simulink model "JulyTestV1"  (Simulink 7.3)
settings: Solver=FixedStepDiscrete  StartTime=0.0  StopTime=inf  FixedStep=0.1  MaxStep=0.2  RelTol=1e-3
libraries: dspmtrx3 x3, simulink x2, vipstatistics x2, dspstat3 x2
(part 1 of 2)
settings Model: Creator=gclayton  LastModifiedBy=wildcat
settings DebuggingCC: InheritedTsInSrcMsg=none
settings RTWCC: SystemTargetFile=rlnx.tlc  GenCodeOnly=on  TemplateMakefile=rlnx_ubuntu.tmf  Description=Linux Real-Time Target  ProcessScript=rlnx_make_rtw_hook
settings RTWCC: CustomInclude=|
  | /usr/local/include/opencv/
  | /usr/local/include/
settings CodeAppCC: GenerateComments=off  SimulinkBlockComments=off
settings STFCustomTargetCC: ModelReferenceCompliant=off  MatFileLogging=on  SystemTargetFile=rlnx.tlc
settings GRTTargetCC: ModelReferenceCompliant=off  ParMdlRefBuildCompliant=off  CompOptLevelCompliant=off
settings CustomProperty: DataType=string  Value="-lm -ldl /usr/local/lib/libopencv_highgui.so.2.4 /usr/local/lib/libopencv_core.so.2.4 /usr/local/lib/libopencv_imgproc.so.2.4  -lc_urg -lc_urg_connection -lc_urg_system -lphidget21"
settings EnumStrPairs: String=PC

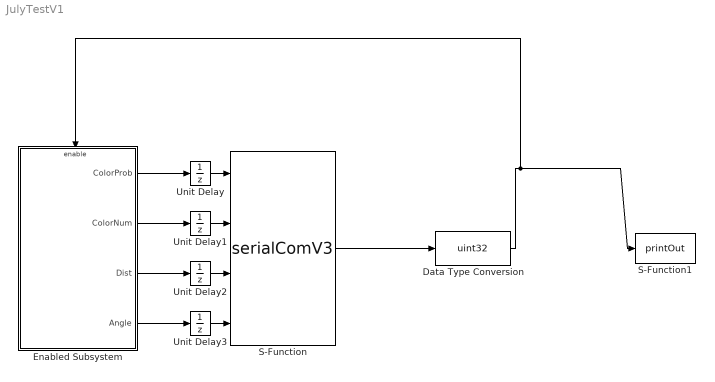
== system JulyTestV1 ==
  Data Type Conversion : DataTypeConversion  OutDataTypeMode=uint32  OutDataType=fixdt(1, 16)  OutScaling=2^0  OutDataTypeStr=uint32
  Enabled Subsystem : Subsystem  TreatAsAtomicUnit=on
  S-Function : S-Function  FunctionName=serialComV3  EnableBusSupport=off
  S-Function1 : S-Function  FunctionName=printOut  EnableBusSupport=off
  Unit Delay : UnitDelay  SampleTime=-1
  Unit Delay1 : UnitDelay  X0=int32(0)  SampleTime=-1
  Unit Delay2 : UnitDelay  X0=int32(0)  SampleTime=-1
  Unit Delay3 : UnitDelay  X0=int32(0)  SampleTime=-1
  wires:
  S-Function/1 -> Data Type Conversion/1
  Data Type Conversion/1 -> S-Function1/1, Enabled Subsystem/Enable
  Enabled Subsystem/1(ColorProb) -> Unit Delay/1
  Enabled Subsystem/2(ColorNum) -> Unit Delay1/1
  Enabled Subsystem/3(Dist) -> Unit Delay2/1
  Enabled Subsystem/4(Angle) -> Unit Delay3/1
  Unit Delay/1 -> S-Function/1
  Unit Delay1/1 -> S-Function/2
  Unit Delay2/1 -> S-Function/3
  Unit Delay3/1 -> S-Function/4

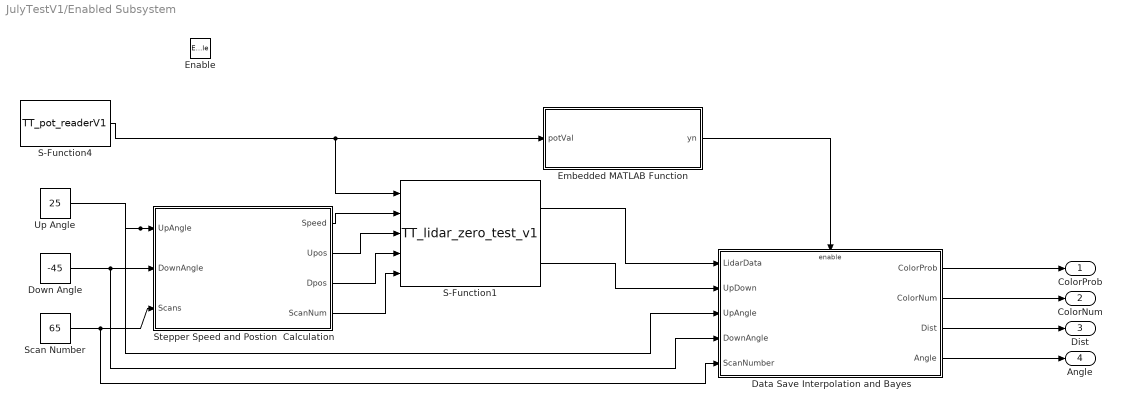
== system JulyTestV1/Enabled Subsystem ==
  Enable : EnablePort
  Data Save Interpolation and Bayes : Subsystem  TreatAsAtomicUnit=on
  Down Angle : Constant  Value=-45  OutDataType=fixdt(1, 16)  OutScaling=2^0
  Embedded MATLAB Function : Stateflow chart
  S-Function1 : S-Function  FunctionName=TT_lidar_zero_test_v1  EnableBusSupport=off
  S-Function4 : S-Function  FunctionName=TT_pot_readerV1  EnableBusSupport=off
  Scan Number : Constant  Value=65  OutDataType=fixdt(1, 16)  OutScaling=2^0
  Stepper Speed and Postion  Calculation : Stateflow chart
  Up Angle : Constant  Value=25  OutDataType=fixdt(1, 16)  OutScaling=2^0
  ColorProb : Outport  OutDataType=fixdt(1, 16)  OutScaling=2^0
  ColorNum : Outport  Port=2  OutDataType=fixdt(1, 16)  OutScaling=2^0
  Dist : Outport  Port=3  OutDataType=fixdt(1, 16)  OutScaling=2^0
  Angle : Outport  Port=4  OutDataType=fixdt(1, 16)  OutScaling=2^0
  wires:
  S-Function4/1 -> S-Function1/1, Embedded MATLAB Function/1(potVal)
  Scan Number/1 -> Stepper Speed and Postion  Calculation/3(Scans), Data Save Interpolation and Bayes/5(ScanNumber)
  Down Angle/1 -> Stepper Speed and Postion  Calculation/2(DownAngle), Data Save Interpolation and Bayes/4(DownAngle)
  Up Angle/1 -> Stepper Speed and Postion  Calculation/1(UpAngle), Data Save Interpolation and Bayes/3(UpAngle)
  Stepper Speed and Postion  Calculation/1(Speed) -> S-Function1/2
  Stepper Speed and Postion  Calculation/2(Upos) -> S-Function1/3
  Stepper Speed and Postion  Calculation/3(Dpos) -> S-Function1/4
  Stepper Speed and Postion  Calculation/4(ScanNum) -> S-Function1/5
  Embedded MATLAB Function/1(yn) -> Data Save Interpolation and Bayes/Enable
  S-Function1/1 -> Data Save Interpolation and Bayes/1(LidarData)
  S-Function1/2 -> Data Save Interpolation and Bayes/2(UpDown)
  Data Save Interpolation and Bayes/1(ColorProb) -> ColorProb/1
  Data Save Interpolation and Bayes/2(ColorNum) -> ColorNum/1
  Data Save Interpolation and Bayes/3(Dist) -> Dist/1
  Data Save Interpolation and Bayes/4(Angle) -> Angle/1

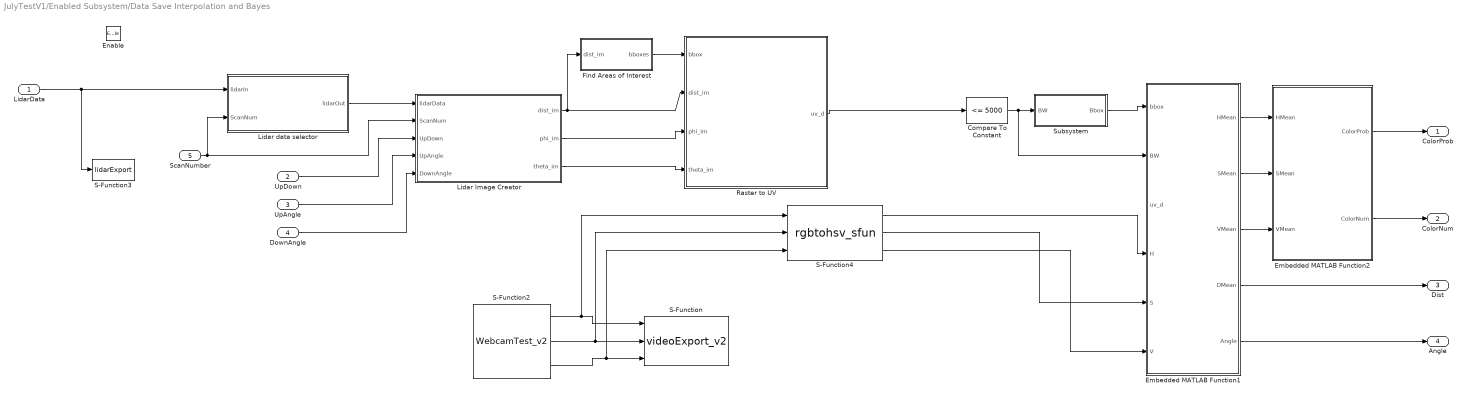
== system JulyTestV1/Enabled Subsystem/Data Save Interpolation and Bayes ==
  LidarData : Inport  OutDataType=fixdt(1, 16)  OutScaling=2^0
  UpDown : Inport  Port=2  OutDataType=fixdt(1, 16)  OutScaling=2^0
  UpAngle : Inport  Port=3  OutDataType=fixdt(1, 16)  OutScaling=2^0
  DownAngle : Inport  Port=4  OutDataType=fixdt(1, 16)  OutScaling=2^0
  ScanNumber : Inport  Port=5  OutDataType=fixdt(1, 16)  OutScaling=2^0
  Enable : EnablePort
  Compare To Constant : simulink/Logic and Bit Operations/Compare To Constant  SystemSampleTime=-1  relop=<=  const=5000  LogicOutDataTypeMode=boolean  ZeroCross=off
  Embedded MATLAB Function1 : Stateflow chart
  Embedded MATLAB Function2 : Stateflow chart
  Find Areas of Interest : Subsystem
  Lidar Image Creator : Stateflow chart
  Lidar data selector : Stateflow chart
  Raster to UV : Stateflow chart
  S-Function : S-Function  FunctionName=videoExport_v2  EnableBusSupport=off
  S-Function2 : S-Function  FunctionName=WebcamTest_v2  EnableBusSupport=off
  S-Function3 : S-Function  FunctionName=lidarExport  EnableBusSupport=off
  S-Function4 : S-Function  FunctionName=rgbtohsv_sfun  EnableBusSupport=off
  Subsystem : Subsystem
  ColorProb : Outport  OutDataType=fixdt(1, 16)  OutScaling=2^0
  ColorNum : Outport  Port=2  OutDataType=fixdt(1, 16)  OutScaling=2^0
  Dist : Outport  Port=3  OutDataType=fixdt(1, 16)  OutScaling=2^0
  Angle : Outport  Port=4  OutDataType=fixdt(1, 16)  OutScaling=2^0
  wires:
  S-Function2/3 -> S-Function/3, S-Function4/3
  S-Function2/2 -> S-Function/2, S-Function4/2
  S-Function2/1 -> S-Function/1, S-Function4/1
  LidarData/1 -> S-Function3/1, Lidar data selector/1(lidarIn)
  ScanNumber/1 -> Lidar data selector/2(ScanNum), Lidar Image Creator/2(ScanNum)
  Lidar data selector/1(lidarOut) -> Lidar Image Creator/1(lidarData)
  UpDown/1 -> Lidar Image Creator/3(UpDown)
  UpAngle/1 -> Lidar Image Creator/4(UpAngle)
  DownAngle/1 -> Lidar Image Creator/5(DownAngle)
  Lidar Image Creator/1(dist_im) -> Raster to UV/2(dist_im), Find Areas of Interest/1(dist_im)
  Lidar Image Creator/2(phi_im) -> Raster to UV/3(phi_im)
  Lidar Image Creator/3(theta_im) -> Raster to UV/4(theta_im)
  Find Areas of Interest/1(bboxes) -> Raster to UV/1(bbox)
  Compare To Constant/1 -> Subsystem/1(BW), Embedded MATLAB Function1/2(BW)
  Subsystem/1(Bbox) -> Embedded MATLAB Function1/1(bbox)
  Embedded MATLAB Function1/3(VMean) -> Embedded MATLAB Function2/3(VMean)
  Embedded MATLAB Function1/2(SMean) -> Embedded MATLAB Function2/2(SMean)
  Embedded MATLAB Function1/1(HMean) -> Embedded MATLAB Function2/1(HMean)
  Raster to UV/1(uv_d) -> Compare To Constant/1
  S-Function4/1 -> Embedded MATLAB Function1/4(H)
  S-Function4/2 -> Embedded MATLAB Function1/5(S)
  S-Function4/3 -> Embedded MATLAB Function1/6(V)
  Embedded MATLAB Function2/1(ColorProb) -> ColorProb/1
  Embedded MATLAB Function2/2(ColorNum) -> ColorNum/1
  Embedded MATLAB Function1/4(DMean) -> Dist/1
  Embedded MATLAB Function1/5(Angle) -> Angle/1

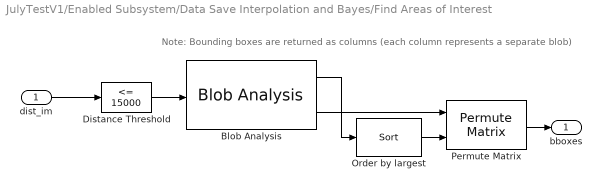
== system JulyTestV1/Enabled Subsystem/Data Save Interpolation and Bayes/Find Areas of Interest ==
  note: Note: Bounding boxes are returned as columns (each column represents a separate blob)
  dist_im : Inport  OutDataType=fixdt(1, 16)  OutScaling=2^0
  Blob Analysis : vipstatistics/Blob Analysis  DialogController=vipDDGCreate  DialogControllerArgs=DataTag0  area=on  centroid=off  bBox=on  majorAxis=off  minorAxis=off  angle=off  eccentricity=off  equivDiameterSq=off  extent=off  perimeter=off  maxBlobs=8  warnIfNumBlobsExceeded=on  isCount=off  useMinArea=off  minArea=0  useMaxArea=off  maxArea=intmax('uint32')  excludeBorderBlob=off  outDT=double  isOutVarDim=off  isFill=on  fillValues=-1  conn=8  isLabel=off  outputMode=Binary point scaling  outputWordLength=32  outputFracLength=16  firstCoeffMode=Binary point scaling  firstCoeffWordLength=16  firstCoeffFracLength=14  secondCoeffMode=Binary point scaling  secondCoeffWordLength=32  secondCoeffFracLength=16  accumMode=Binary point scaling  accumWordLength=32  accumFracLength=0  prodOutputMode=Binary point scaling  prodOutputWordLength=32  prodOutputFracLength=16  roundingMode=Floor  overflowMode=off
  Distance Threshold : simulink/Logic and Bit Operations/Compare To Constant  SystemSampleTime=-1  relop=<=  const=15000  LogicOutDataTypeMode=boolean  ZeroCross=off
  Order by largest : dspstat3/Sort  DialogController=dspDDGCreate  DialogControllerArgs=DataTag1  otype=Index  dir=Descending  sortAlg=Quick sort  roundingMode=Floor  overflowMode=off
  Permute Matrix : dspmtrx3/Permute Matrix  mode=Columns  ZeroOneIdxMode=One-based  errmode=Clip index  checkDims=off
  bboxes : Outport  OutDataType=fixdt(1, 16)  OutScaling=2^0
  wires:
  dist_im/1 -> Distance Threshold/1
  Distance Threshold/1 -> Blob Analysis/1
  Blob Analysis/2 -> Permute Matrix/1
  Order by largest/1 -> Permute Matrix/2
  Blob Analysis/1 -> Order by largest/1
  Permute Matrix/1 -> bboxes/1

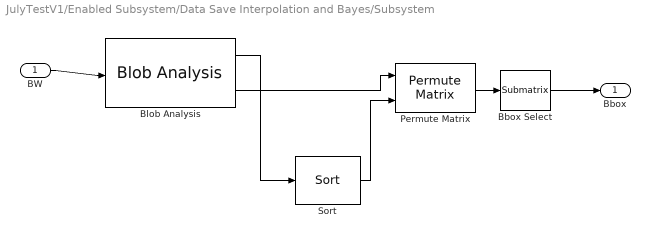
== system JulyTestV1/Enabled Subsystem/Data Save Interpolation and Bayes/Subsystem ==
  BW : Inport  OutDataType=fixdt(1, 16)  OutScaling=2^0
  Bbox Select : dspmtrx3/Submatrix  RowSpan=One row  RowStartMode=First  RowStartIndex=1  RowEndMode=Last  RowEndIndex=1  ColSpan=All columns  ColStartMode=First  ColStartIndex=1  ColEndMode=Last  ColEndIndex=1
  Blob Analysis : vipstatistics/Blob Analysis  DialogController=vipDDGCreate  DialogControllerArgs=DataTag2  area=on  centroid=off  bBox=on  majorAxis=off  minorAxis=off  angle=off  eccentricity=off  equivDiameterSq=off  extent=off  perimeter=off  maxBlobs=20  warnIfNumBlobsExceeded=on  isCount=off  useMinArea=on  minArea=20  useMaxArea=off  maxArea=intmax('uint32')  excludeBorderBlob=off  outDT=double  isOutVarDim=off  isFill=on  fillValues=-1  conn=8  isLabel=off  outputMode=Binary point scaling  outputWordLength=32  outputFracLength=16  firstCoeffMode=Binary point scaling  firstCoeffWordLength=16  firstCoeffFracLength=14  secondCoeffMode=Binary point scaling  secondCoeffWordLength=32  secondCoeffFracLength=16  accumMode=Binary point scaling  accumWordLength=32  accumFracLength=0  prodOutputMode=Binary point scaling  prodOutputWordLength=32  prodOutputFracLength=16  roundingMode=Floor  overflowMode=off
  Permute Matrix : dspmtrx3/Permute Matrix  mode=Columns  ZeroOneIdxMode=One-based  errmode=Clip index  checkDims=off
  Sort : dspstat3/Sort  DialogController=dspDDGCreate  DialogControllerArgs=DataTag3  otype=Index  dir=Descending  sortAlg=Quick sort  roundingMode=Floor  overflowMode=off
  Bbox : Outport  OutDataType=fixdt(1, 16)  OutScaling=2^0
  wires:
  BW/1 -> Blob Analysis/1
  Blob Analysis/1 -> Sort/1
  Sort/1 -> Permute Matrix/2
  Blob Analysis/2 -> Permute Matrix/1
  Permute Matrix/1 -> Bbox Select/1
  Bbox Select/1 -> Bbox/1

== matlab function Enabled Subsystem/Stepper Speed and Postion Calculation ==
  data: UpAngle input double; Speed output double; DownAngle input double; Scans input double; Upos output double; Dpos output double; ScanNum output double
function [Speed,Upos,Dpos,ScanNum] = stepper_calc(UpAngle,DownAngle,Scans)

% This function inputs desired positive and negative scan angles
% and desired number of scans and outputs results positions for
% the stepper and the required speed of the stepper motor to properly
% move so the desired number of scans is obtained over the course of
% the motion of the stepper

% Scan Number requires no change
ScanNum = Scans;

% Transformation of angle to stepper position obtained from stepper calibration
% Output must be an integer
% 57 is added or subtracted due to wobble of gimbal system
Upos = round(UpAngle*1036/45)-57;
Dpos = round(DownAngle*1036/45)+57;

% Transformation of speed based 
% Output must be an interger
Speed = round(abs(UpAngle-DownAngle) * (1214/90) * 65/Scans);

== matlab function Enabled Subsystem/Embedded MATLAB Function ==
  data: potVal input double; yn output double
function yn = check_pot_val(potVal)
%#eml

% Pot value may initially be zero.
% Check for this and output a 1 or zero to 
% control whether the rest of model runs
if (potVal == 0)
    yn = 0;
else
    yn = 1;
end

== matlab function Enabled Subsystem/Data Save Interpolation and Bayes/Lidar data selector ==
  data: lidarIn input double; lidarOut output double; ScanNum input double
function lidarOut = data_selector(lidarIn,ScanNum)
% Lidar data is always input as a 1x70200 matrix.
% If Scan Number is less than 65 some of this data may be blank
% Select only the parts of the matrix where data has been collected

% FullLength = 1080*65;
% DataLength =  1080*ScanNum;
% lidarOut = zeros(1,FullLength);

ClosePts = (lidarIn < 3);
lidarOut = lidarIn + 30000*ClosePts;

% for i = 1:DataLength
%     if (lidarIn(i) < 3)
%         lidarIn(i) = 30000;
%     end
%     lidarOut(i) = lidarIn(i);
% end

%lidarOut = lidarIn(1,1:DataLength);

== matlab function Enabled Subsystem/Data Save Interpolation and Bayes/Lidar Image Creator ==
  data: lidarData input double; ScanNum input double; dist_im output double; phi_im output double; theta_im output double; UpDown input double; UpAngle input double; DownAngle input double
function [dist_im, phi_im, theta_im] = image_creator(lidarData,ScanNum,UpDown,UpAngle,DownAngle)
%#eml

% Define variables based on gimbal system and scan pattern
FullLength = 1080*65;
DataLength = 1080*ScanNum;
h = 36.3;

% Define Data sizes
phim = zeros(1,FullLength);
thetam = zeros(1,FullLength);
distm = zeros(1,FullLength);
dist_im = zeros(65,540);
phi_im = zeros(65,540);
theta_im = zeros(65,540);


%Define phi_rad: angles corresponding to one lidar scan
l = 1:1080;
phi_rad = (-45 + 0.25*l)*pi/180;

% Repeat phim for number of scans
for i = 1:ScanNum
        
    for j = 1 : 1080
        phi_val = 1080*(i-1) + j;
        phim(1,phi_val) = phi_rad(1,j);
    end
end

% Theta changes from -45 to 45 degrees over the duration of the scan
theta_min = DownAngle*pi/180;
theta_max = UpAngle*pi/180;
theta_step = (theta_max - theta_min)/DataLength;

for i1 = 1:DataLength
    if (UpDown == 0)
        thetam(i1) = theta_max - theta_step*(i1-1);
    elseif (UpDown == 1)
        thetam(i1) = theta_min + theta_step*(i1-1);
    end
end

% Distance matrix is directly from lidar data
distm = lidarData';


% Create images for distance, phi, and theta
for i2 = 1:ScanNum
    for j2 = 1:540
        dist_im(i2,j2) = distm(1, 270+j2 + 1080*(i2-1));
        phi_im(i2,j2) = phim(1, 270+j2 + 1080*(i2-1));
        theta_im(i2,j2) = thetam(1, 270+j2 + 1080*(i2-1));
    end
    
end

== matlab function Enabled Subsystem/Data Save Interpolation and Bayes/Raster to UV ==
  data: bbox input double; uv_d output double; dist_im input double; phi_im input double; theta_im input double
function uv_d  = fcn(bbox,dist_im,phi_im,theta_im)
% Written by Anderson Lebbad on July 3, 2014
% Last Edited:
%
% This function transforms the lidar raster image into u,v coordinates,
% with an xyz transformation and change of perspective from the lidar to
% the camera

%% Set Variables

% Find the number of valid bounding boxes
numBBox = 8 - sum(bbox(1,:) == -1);

beyondRange = 30000;
uv_d = beyondRange*ones(480,640);

% Initialize size of X,Y and Z matrices
X = zeros(size(dist_im));
Y = zeros(size(dist_im));
Z = zeros(size(dist_im));
Xc = zeros(size(dist_im));
Yc = zeros(size(dist_im));
Zc = zeros(size(dist_im));
Xn = zeros(size(dist_im));
Yn = zeros(size(dist_im));
Xp = zeros(size(dist_im));
Yp = zeros(size(dist_im));
Dp = zeros(size(dist_im));
r2 = zeros(size(dist_im));
r6 = zeros(size(dist_im));
Xd = zeros(size(dist_im));
Yd = zeros(size(dist_im));

% Height of the lidar on the gimbal
h = 36.3;

% Translation vector (in millimeters)
t = [24; -113; 38];

% Rotation angles
phi = (-90+6)*pi/180;
theta = 0*pi/180;

% Rotation about the x-axis
Rx = [1 0 0; 0 cos(phi) sin(phi); 0 -sin(phi) cos(phi)];
% Followed by rotation about the y-axis
R = [cos(theta) 0 -sin(theta); 0 1 0; sin(theta) 0 cos(theta)]*Rx;

% Transformation matrix
T = [R t];

% Radial Distortions
RadDist = [0.069102182282360,-0.154608606024690,0.020241053576861];

% Intrinsic Matrix
K = [5.548581600685270e+02,0,0;0,5.523116000564020e+02,0;3.135858904821101e+02,2.190392333699872e+02,1];
KK = K';

% Iterate filling points into XYZ matrices for each valid bbox
for i = 1:numBBox
    
    % Initialize values for looped info
    minXp = 10000;
    maxXp = -10000;
    minYp = 10000;
    maxYp = -10000;
    
    % Find region to fill
    minX = bbox(1,i);
    maxX = minX + bbox(3,i) - 1;
    minY = bbox(2,i);
    maxY = minY + bbox(4,i) - 1;
    
    % Loop for each pixel in the bounding box
    for j = minX:maxX
        for k = minY:maxY
            % Convert to XYZ
            X(k,j) = dist_im(k,j).*cos(phi_im(k,j));
            Y(k,j) = dist_im(k,j).*sin(phi_im(k,j)).*cos(theta_im(k,j))-h.*sin(theta_im(k,j));
            Z(k,j) = dist_im(k,j).*sin(phi_im(k,j)).*sin(theta_im(k,j))+h.*cos(theta_im(k,j));
            
            % Transformation to camera coordinate frame
            Xc(k,j) = T(1,1)*X(k,j)+T(1,2)*Y(k,j)+T(1,3)*Z(k,j)+T(1,4);
            Yc(k,j) = T(2,1)*X(k,j)+T(2,2)*Y(k,j)+T(2,3)*Z(k,j)+T(2,4);
            Zc(k,j) = T(3,1)*X(k,j)+T(3,2)*Y(k,j)+T(3,3)*Z(k,j)+T(3,4);
            
            % Normalize Coordinates
            Xn(k,j) = Xc(k,j)./Zc(k,j);
            Yn(k,j) = Yc(k,j)./Zc(k,j);
            
            % Calculate Distance to each point from camera
            Dp(k,j) = sqrt(Xc(k,j).^2+Yc(k,j).^2+Zc(k,j).^2);
            
            % Radial Vectors
            r2(k,j) = Xn(k,j).^2+Yn(k,j).^2;
            r6(k,j) = r2(k,j).^3;
            
            % Distorted Coodinates
            Xd(k,j) = Xn(k,j).*(1+RadDist(1).*r2(k,j)+RadDist(3).*r6(k,j));
            Yd(k,j) = Yn(k,j).*(1+RadDist(1).*r2(k,j)+RadDist(3).*r6(k,j));
            
            % Pixel Coordinates
            Xp(k,j) = KK(1,1)*Xd(k,j)+KK(1,2)*Yd(k,j)+KK(1,3);
            Yp(k,j) = KK(2,1)*Xd(k,j)+KK(2,2)*Yd(k,j)+KK(2,3);
            
            % Find area the blob is bound by in the image coordinates
            minXp = ceil(min(Xp(k,j),minXp));
            maxXp = floor(max(Xp(k,j),maxXp));
            minYp = ceil(min(Yp(k,j),minYp));
            maxYp = floor(max(Yp(k,j),maxYp));
        end
    end
    
    % Check to make sure blob is (at least partially) within image frame
    if (minXp < 640) && (maxXp > 1) && (minYp < 480) && (maxYp > 1)
        
        % Set interpolation vectors to not exceed frame
        minXp = max(minXp,1);
        maxXp = min(maxXp,640);
        minYp = max(minYp,1);
        maxYp = min(maxYp,480);
        
        % Run interpolation over bounded region
        for j3 = minXp:maxXp
            for k3 = minYp:maxYp
                
                % Initialize values
                l1normSmall = 1000;
                uPt = int32(1);
                vPt = int32(1);
                
                % Loop for each pixel in original bounding box
                for j2 = minX:maxX
                    for k2 = minY:maxY
                        
                        % L1 Norm for nearest neighbor interpolation
                        l1norm = abs(Xp(k2,j2)-j3)+abs(Yp(k2,j2)-k3);
                        
                        % Check against previously smallest L1 norm
                        if l1norm < l1normSmall
                            % Replace previous value with current value
                            l1normSmall = l1norm;
                            uPt = j2;
                            vPt = k2;
                        end
                    end
                end
                
                % Use pointer array to assign depth values into output frame
                uv_d(k3,j3) = Dp(uPt,vPt);
                
            end
        end
    end
end

end

== matlab function Enabled Subsystem/Data Save Interpolation and Bayes/Embedded MATLAB Function1 ==
  data: bbox input double; HMean output double; BW input double; uv_d input double; H input double; S input double; V input double; SMean output double; VMean output double; DMean output double; Angle output double
function [HMean, SMean, VMean, DMean, Angle] = bbox_hist(bbox, BW, uv_d, H, S, V)
%This function creates a histogram of the color region of a detected object
%identified in a binary image within a bounding box

%Initialize variables
pixels = 0;
DRunAve = 0;
HRunAve = 0;
SRunAve = 0;
VRunAve = 0;
FoV = 62;

%Parse bbox data
left = bbox(1);
right = left + bbox(3) - 1;
bottom = bbox(2);
top = bottom + bbox(4) - 1;
Angle = int32((left + bbox(3)/2-320)/320*FoV/2);

%Check to see if valid bbox is found
if left~=-1
    %Scan the detected region of the binary image and generate histograms
    for j=left:right
        for i=bottom:top
            if BW(i,j) == 1
                pixels = pixels + 1;
                DRunAve = ((pixels-1)/pixels)*DRunAve + (1/pixels)*double(uv_d(i,j));
                HRunAve = ((pixels-1)/pixels)*HRunAve + (1/pixels)*double(H(i,j));
                SRunAve = ((pixels-1)/pixels)*SRunAve + (1/pixels)*double(S(i,j));
                VRunAve = ((pixels-1)/pixels)*VRunAve + (1/pixels)*double(V(i,j));
            end
        end
    end
end

%Means must be integers to use in Bayes Filter
DMean = int32(DRunAve);
HMean = uint8(HRunAve);
SMean = uint8(SRunAve);
VMean = uint8(VRunAve);

end
